simulink model "sampleModel148"  (R2021b)
settings: Solver=VariableStepAuto  StartTime=0.0  StopTime=10.0  RelTol=1e-3
libraries: simulink x4
settings Model: Creator=user  LastModifiedBy=user

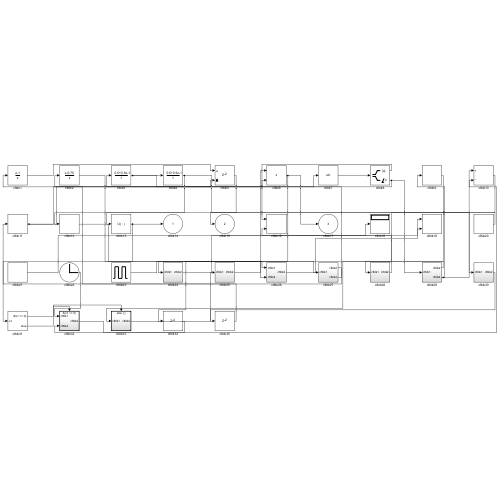
[thumbnail: Simulink's stored preview of the top-level diagram]
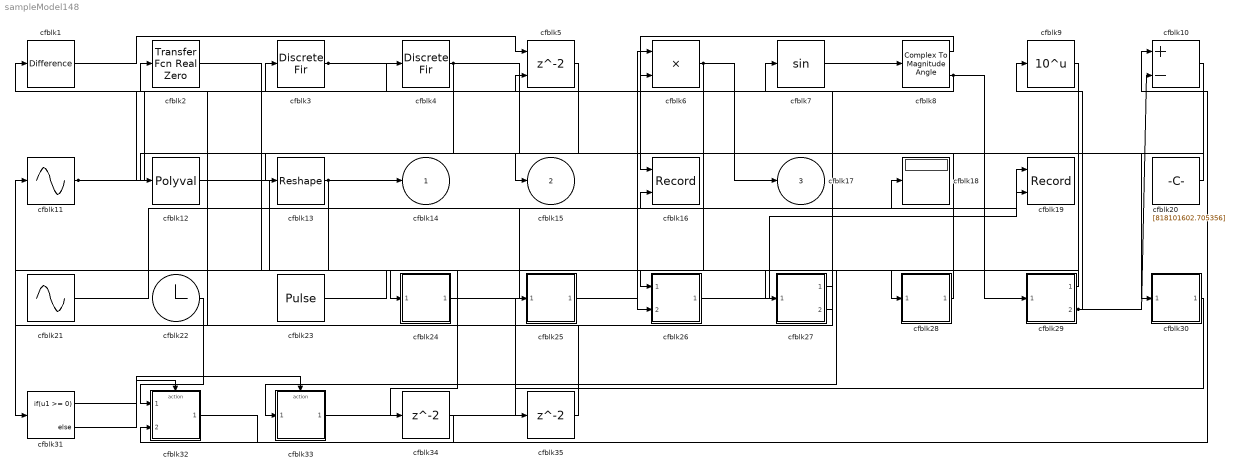
== system sampleModel148 ==
  cfblk1 : simulink/Discrete/Difference  ICPrevInput=0.0  OutMin=[]  OutMax=[]  OutDataTypeStr=Inherit: Inherit via back propagation  OutDataType=fixdt(1, 16)  OutScaling=2^-10  DoSatur=off
  cfblk10 : Sum  Inputs=+-
  cfblk11 : Sin  TimeSource=Use external signal  SampleTime=0
  cfblk12 : Polyval  Coefs=[ +2.081618890e-019, -1.441693666e-014, +4.719686976e-010, -8.536869453e-006, +1.621573104e-001, -8.087801117e+001 ]
  cfblk13 : Reshape
  cfblk16 : Record  FileSettingsInternal="{\"entries\":[{\"content\":{\"excelSettings\":{\"content\":{},\"type\":\"Streamout.ExcelSettings\"}},\"type\":\"Streamout.FileSettingStorage\",\"uuid\":\"b027f13b-7ca7-49e6-b85d-a561881e7aea\"}],\"packageUris\":[\"http://schema.mathworks.com/mf0/streamout_blocks/R2020a\"],\"version\":\"1.0\"}"  Layout=[1 1]  SignalsInternal="{\"entries\":[{\"content\":{\"signals\":[{\"content\":{\"blockPath\":[\"sampleModel148/cfblk16\"],\"channel\":[],\"dimensions\":[1],\"domain\":\"sampleModel148/cfblk16\",\"lineColor\":\"#a2142f\",\"plots\":[1],\"port\":1,\"sid\":[\"\"],\"signalID\":5356,\"signalName\":\"cfblk8:1\"},\"type\":\"RecordBlkView.Signal\",\"uuid\":\"ed710109-99ea-47aa-aeca-7e9a823f4830\"},{\"content\":{\"blockPath\":[\"sampleModel148/cfblk16\"],\"channel\":[],\"dimensions\":[1],\"domain\":\"sampleModel148/cfblk16\",\"lineColor\":\"#139fff\",\"plots\":[1],\"port\":2,\"sid\":[\"\"],\"signalID\":5360,\"signalName\":\"cfblk28\"},\"type\":\"RecordBlkView.Signal\",\"uuid\":\"239f5b95-602e-4f61-bb3f-210a9afe290f\"}]},\"type\":\"RecordBlkView.InputSignals\",\"uuid\":\"2c01184d-9629-409b-aeb1-b862b603ea59\"}],\"packageUris\":[\"http://schema.mathworks.com/mf0/streamout_blocks/R2020a\"],\"version\":\"1.0\"}"  VisualizationBindings="{\"xyplotplugin\":{\"info\":[{\"series\":[{\"bindingParametersList\":[{\"parameter\":\"X-Axis\",\"signalID\":5356,\"signalName\":\"cfblk8:1\"},{\"parameter\":\"Y-Axis\",\"signalID\":5360,\"signalName\":\"cfblk28\"}],\"seriesID\":20638}],\"subplotID\":1}]}}"  CompatibilityTag=XY
  cfblk18 : Display
  cfblk19 : Record  FileSettingsInternal="{\"entries\":[{\"content\":{\"excelSettings\":{\"content\":{},\"type\":\"Streamout.ExcelSettings\"}},\"type\":\"Streamout.FileSettingStorage\",\"uuid\":\"d953e4ab-c191-438b-b4c1-9475d4502db0\"}],\"packageUris\":[\"http://schema.mathworks.com/mf0/streamout_blocks/R2020a\"],\"version\":\"1.0\"}"  Layout=[1 1]  SignalsInternal="{\"entries\":[{\"content\":{\"signals\":[{\"content\":{\"blockPath\":[\"sampleModel148/cfblk19\"],\"channel\":[],\"dimensions\":[1],\"domain\":\"sampleModel148/cfblk19\",\"lineColor\":\"#a2142f\",\"plots\":[1],\"port\":1,\"sid\":[\"\"],\"signalID\":5364,\"signalName\":\"cfblk26\"},\"type\":\"RecordBlkView.Signal\",\"uuid\":\"680231d5-d346-436f-ba17-d46778f7a71e\"},{\"content\":{\"blockPath\":[\"sampleModel148/cfblk19\"],\"channel\":[],\"dimensions\":[1],\"domain\":\"sampleModel148/cfblk19\",\"lineColor\":\"#139fff\",\"plots\":[1],\"port\":2,\"sid\":[\"\"],\"signalID\":5368,\"signalName\":\"cfblk24\"},\"type\":\"RecordBlkView.Signal\",\"uuid\":\"aa3e67de-9c9e-412d-82bc-d20d43b8d491\"}]},\"type\":\"RecordBlkView.InputSignals\",\"uuid\":\"651ab1f4-4682-4293-806f-abddeb1a3a0e\"}],\"packageUris\":[\"http://schema.mathworks.com/mf0/streamout_blocks/R2020a\"],\"version\":\"1.0\"}"  VisualizationBindings="{\"xyplotplugin\":{\"info\":[{\"series\":[{\"bindingParametersList\":[{\"parameter\":\"X-Axis\",\"signalID\":5364,\"signalName\":\"cfblk26\"},{\"parameter\":\"Y-Axis\",\"signalID\":5368,\"signalName\":\"cfblk24\"}],\"seriesID\":17137}],\"subplotID\":1}]}}"  CompatibilityTag=XY
  cfblk2 : simulink/Discrete/Transfer Fcn Real Zero  ZeroZ=0.75  ICPrevInput=0.0  DoSatur=off
      settings: SourceProductBaseCode=SL
  cfblk20 : Constant  Value=[818101602.705356]  SampleTime=1
  cfblk21 : Sin  Amplitude=[-182354528.104471]  Bias=[-693142871.080695]  SampleTime=0
  cfblk22 : Clock
  cfblk23 : DiscretePulseGenerator  PulseType=Time based  Amplitude=[879322730.329937]  Period=[72538017.737468]  PulseWidth=5  PhaseDelay=[7.000000]
  cfblk24 : Subsystem
  cfblk25 : Subsystem
  cfblk26 : Subsystem
  cfblk27 : Subsystem
  cfblk28 : Subsystem
  cfblk29 : Subsystem
  cfblk3 : DiscreteFir  SampleTime=1
  cfblk30 : Subsystem
  cfblk31 : If  IfExpression=u1 >= 0  SampleTime=1
  cfblk32 : Subsystem  TreatAsAtomicUnit=on
  cfblk33 : Subsystem  TreatAsAtomicUnit=on
  cfblk34 : Delay  SampleTime=1
  cfblk35 : Delay  SampleTime=1
  cfblk4 : DiscreteFir  SampleTime=1
  cfblk5 : Delay  ShowEnablePort=on  SampleTime=1
      settings: InputPortMap=u0,e6
  cfblk6 : Product  Inputs=**
  cfblk7 : Trigonometry
  cfblk8 : ComplexToMagnitudeAngle
  cfblk9 : Math  Operator=10^u  SaturateOnIntegerOverflow=on
  cfblk14 : Outport
  cfblk15 : Outport  Port=2
  cfblk17 : Outport  Port=3
  wires:
  cfblk21/1 -> cfblk18/1
  cfblk27/1(cfblk2) -> cfblk11/1
  cfblk6/1 -> cfblk17/1, cfblk34/1
  cfblk9/1 -> cfblk33/1(cfblk1)
  cfblk26/1(cfblk2) -> cfblk19/1
  cfblk24/1(cfblk2) -> cfblk19/2
  cfblk8/1 -> cfblk16/1
  cfblk33/1(cfblk2) -> cfblk25/1(cfblk1)
  cfblk3/1 -> cfblk4/1, cfblk5/2
  cfblk32/1(cfblk2) -> cfblk10/1
  cfblk11/1 -> cfblk7/1, cfblk6/2
  cfblk10/1 -> cfblk28/1(cfblk1)
  cfblk29/1(cfblk2) -> cfblk24/1(cfblk1)
  cfblk27/2(cfblk4) -> cfblk3/1
  cfblk8/2 -> cfblk1/1, cfblk29/1(cfblk1)
  cfblk2/1 -> cfblk27/1(cfblk1)
  cfblk13/1 -> cfblk31/1, cfblk14/1
  cfblk23/1 -> cfblk26/1(cfblk1)
  cfblk1/1 -> cfblk5/1
  cfblk29/2(cfblk4) -> cfblk10/2, cfblk9/1
  cfblk22/1 -> cfblk32/1(cfblk1)
  cfblk20/1 -> cfblk15/1
  cfblk4/1 -> cfblk30/1(cfblk1), cfblk13/1
  cfblk5/1 -> cfblk12/1
  cfblk28/1(cfblk2) -> cfblk16/2
  cfblk12/1 -> cfblk26/2(cfblk4)
  cfblk7/1 -> cfblk8/1
  cfblk25/1(cfblk2) -> cfblk6/1
  cfblk31/1 -> cfblk32/Action
  cfblk31/2 -> cfblk33/Action
  cfblk34/1 -> cfblk32/2(cfblk4)
  cfblk30/1(cfblk2) -> cfblk35/1
  cfblk35/1 -> cfblk2/1

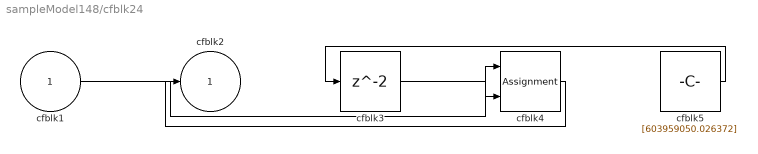
== system sampleModel148/cfblk24 ==
  cfblk1 : Inport
  cfblk3 : Delay  SampleTime=1
  cfblk4 : Assignment  DiagnosticForDimensions=Warning  IndexOptions=Index vector (dialog)  Indices=1  OutputSizes=1
  cfblk5 : Constant  Value=[603959050.026372]  SampleTime=1
  cfblk2 : Outport
  wires:
  cfblk5/1 -> cfblk3/1
  cfblk1/1 -> cfblk4/1
  cfblk3/1 -> cfblk4/2
  cfblk4/1 -> cfblk2/1

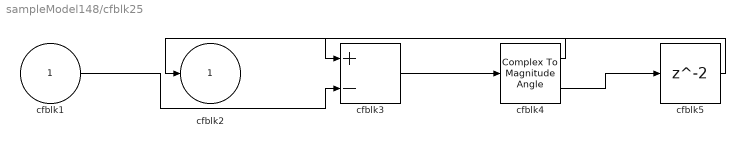
== system sampleModel148/cfblk25 ==
  cfblk1 : Inport
  cfblk3 : Sum  Inputs=+-
  cfblk4 : ComplexToMagnitudeAngle
  cfblk5 : Delay  SampleTime=1
  cfblk2 : Outport
  wires:
  cfblk3/1 -> cfblk4/1
  cfblk4/1 -> cfblk2/1
  cfblk1/1 -> cfblk3/2
  cfblk4/2 -> cfblk5/1
  cfblk5/1 -> cfblk3/1

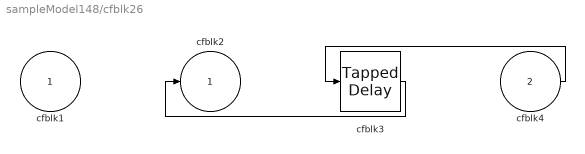
== system sampleModel148/cfblk26 ==
  cfblk1 : Inport
  cfblk4 : Inport  Port=2
  cfblk3 : simulink/Discrete/Tapped Delay  vinit=0.0  samptime=-1  NumDelays=1  DelayOrder=Oldest  includeCurrent=off
  cfblk2 : Outport
  wires:
  cfblk4/1 -> cfblk3/1
  cfblk3/1 -> cfblk2/1

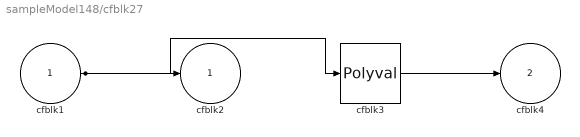
== system sampleModel148/cfblk27 ==
  cfblk1 : Inport
  cfblk3 : Polyval  Coefs=[ +2.081618890e-019, -1.441693666e-014, +4.719686976e-010, -8.536869453e-006, +1.621573104e-001, -8.087801117e+001 ]
  cfblk2 : Outport
  cfblk4 : Outport  Port=2
  wires:
  cfblk1/1 -> cfblk3/1, cfblk2/1
  cfblk3/1 -> cfblk4/1

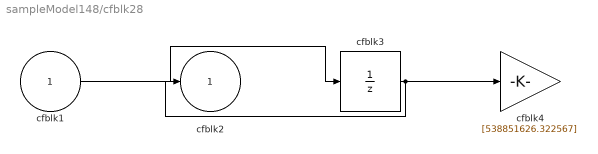
== system sampleModel148/cfblk28 ==
  cfblk1 : Inport
  cfblk3 : UnitDelay  HasFrameUpgradeWarning=on
  cfblk4 : Gain  Gain=[538851626.322567]
  cfblk2 : Outport
  wires:
  cfblk1/1 -> cfblk3/1
  cfblk3/1 -> cfblk2/1, cfblk4/1

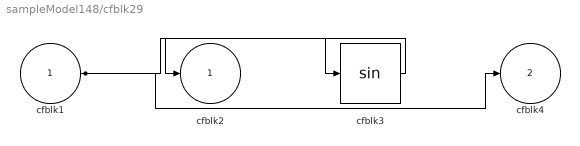
== system sampleModel148/cfblk29 ==
  cfblk1 : Inport
  cfblk3 : Trigonometry
  cfblk2 : Outport
  cfblk4 : Outport  Port=2
  wires:
  cfblk3/1 -> cfblk2/1
  cfblk1/1 -> cfblk4/1, cfblk3/1

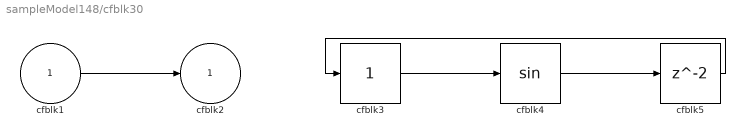
== system sampleModel148/cfblk30 ==
  cfblk1 : Inport
  cfblk3 : simulink/Math Operations/Slider Gain  gain=1  low=0  high=2
  cfblk4 : Trigonometry
  cfblk5 : Delay  SampleTime=1
  cfblk2 : Outport
  wires:
  cfblk1/1 -> cfblk2/1
  cfblk3/1 -> cfblk4/1
  cfblk4/1 -> cfblk5/1
  cfblk5/1 -> cfblk3/1

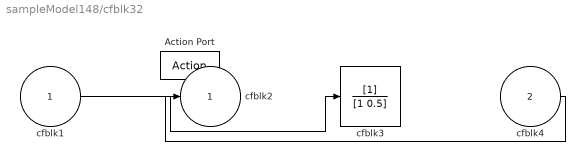
== system sampleModel148/cfblk32 ==
  cfblk1 : Inport
  cfblk4 : Inport  Port=2
  Action Port : ActionPort  ActionPortLabel=if(u1 >= 0)
  cfblk3 : DiscreteFilter
  cfblk2 : Outport
  wires:
  cfblk1/1 -> cfblk3/1
  cfblk4/1 -> cfblk2/1

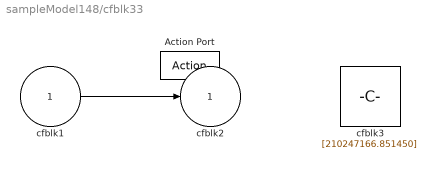
== system sampleModel148/cfblk33 ==
  cfblk1 : Inport
  Action Port : ActionPort  ActionPortLabel=else
  cfblk3 : Constant  Value=[210247166.851450]  SampleTime=1
  cfblk2 : Outport
  wires:
  cfblk1/1 -> cfblk2/1
